simulink model "SunSol_mathBlock"  (R2025b)
settings: Solver=VariableStepAuto  StartTime=0.0  StopTime=10.0  RelTol=1e-3
settings Model: Creator=Abdulwahid  LastModifiedBy=Abdulwahid
settings DataIOCC: SaveOutput=off  SignalLogging=off

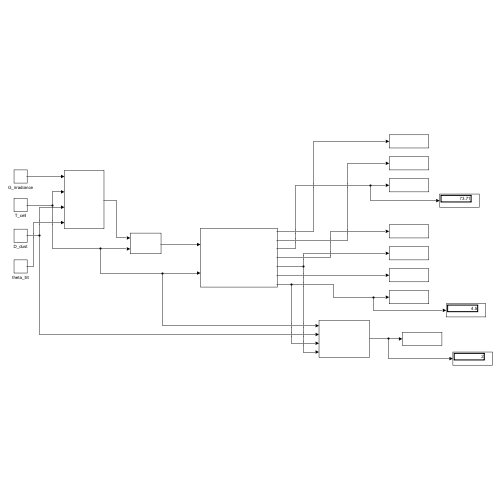
[thumbnail: Simulink's stored preview of the top-level diagram]
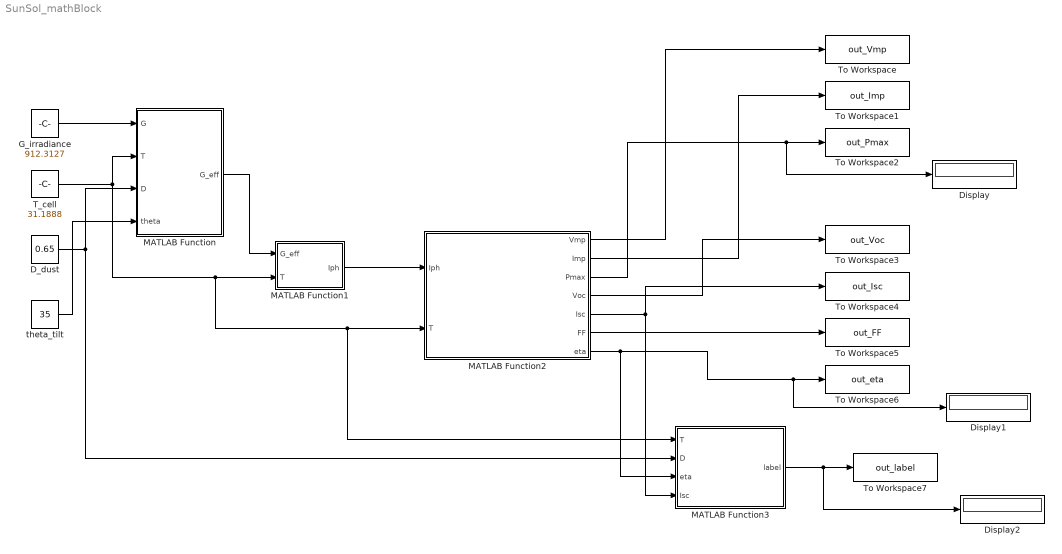
== system SunSol_mathBlock ==
  D_dust : Constant  Value=0.65
  Display : Display
  Display1 : Display
  Display2 : Display
  G_irradiance : Constant  Value=912.3127
  MATLAB Function : MATLAB Function  TreatAsAtomicUnit=on
  MATLAB Function1 : MATLAB Function  TreatAsAtomicUnit=on
  MATLAB Function2 : MATLAB Function  TreatAsAtomicUnit=on
  MATLAB Function3 : MATLAB Function  TreatAsAtomicUnit=on
  T_cell : Constant  Value=31.1888
  To Workspace : ToWorkspace  VariableName=out_Vmp  SampleTime=-1
  To Workspace1 : ToWorkspace  VariableName=out_Imp  SampleTime=-1
  To Workspace2 : ToWorkspace  VariableName=out_Pmax  SampleTime=-1
  To Workspace3 : ToWorkspace  VariableName=out_Voc  SaveFormat=Timeseries  SampleTime=-1
  To Workspace4 : ToWorkspace  VariableName=out_Isc  SampleTime=-1
  To Workspace5 : ToWorkspace  VariableName=out_FF  SampleTime=-1
  To Workspace6 : ToWorkspace  VariableName=out_eta  SampleTime=-1
  To Workspace7 : ToWorkspace  VariableName=out_label  SampleTime=-1
  theta_tilt : Constant  Value=35
  wires:
  G_irradiance/1 -> MATLAB Function/1(G)
  T_cell/1 -> MATLAB Function/2(T), MATLAB Function3/1(T), MATLAB Function2/2(T), MATLAB Function1/2(T)
  MATLAB Function/1(G_eff) -> MATLAB Function1/1(G_eff)
  MATLAB Function1/1(Iph) -> MATLAB Function2/1(Iph)
  MATLAB Function2/1(Vmp) -> To Workspace/1
  MATLAB Function2/2(Imp) -> To Workspace1/1
  MATLAB Function2/3(Pmax) -> Display/1, To Workspace2/1
  MATLAB Function2/4(Voc) -> To Workspace3/1
  MATLAB Function2/5(Isc) -> MATLAB Function3/4(Isc), To Workspace4/1
  MATLAB Function2/6(FF) -> To Workspace5/1
  MATLAB Function2/7(eta) -> MATLAB Function3/3(eta), Display1/1, To Workspace6/1
  MATLAB Function3/1(label) -> Display2/1, To Workspace7/1
  D_dust/1 -> MATLAB Function/3(D), MATLAB Function3/2(D)
  theta_tilt/1 -> MATLAB Function/4(theta)

== matlab function SunSol_mathBlock/MATLAB Function1 ==
  data: G_eff input; Iph output; T input
function Iph = calc_Iph(G_eff, T)
    Isc_ref = 8.91;
    Ki      = 0.0032;
    G_ref   = 1000;
    T_ref   = 25;
    Iph = (Isc_ref + Ki .* (T - T_ref)) .* (G_eff ./ G_ref);
end

== matlab function SunSol_mathBlock/MATLAB Function ==
  data: G input; G_eff output; T input; D input; theta input
function G_eff = calc_Geff(G, T, D, theta)
    G_eff = G .* cosd(theta) .* (1 - D);
end

== matlab function SunSol_mathBlock/MATLAB Function2 ==
  data: Iph input; Vmp output; T input; Imp output; Pmax output; Voc output; Isc output; FF output; eta output
function [Vmp,Imp,Pmax,Voc,Isc,FF,eta] = solve_IV(Iph, T)
    q=1.602e-19; k=1.381e-23; n=1.3;
    A=1.638; Rs=0.221; Rsh=415.405; Ns=60;
    T_ref=25; Kv=-0.0023;
    Tc = T + 273.15;
    Vt = (n*k*Tc*Ns)/q;
    I0_ref = 2.0716e-9;
    I0 = I0_ref*(Tc/(T_ref+273.15))^3 ...
         *exp((q*1.12)/(n*k)*(1/(T_ref+273.15)-1/Tc));
    Voc = Ns*(Vt*log(Iph/I0+1)) + Kv*(T-T_ref);
    Isc = Iph;
    V_arr = linspace(0,Voc,500);
    I_arr = zeros(1,500);
    for i=1:500
        V=V_arr(i); I=Iph;
        for j=1:50
            F  = I-Iph+I0*(exp((V+I*Rs)/Vt)-1)+(V+I*Rs)/Rsh;
            dF = 1+I0*(Rs/Vt)*exp((V+I*Rs)/Vt)+Rs/Rsh;
            I  = I - F/dF;
        end
        I_arr(i)=max(I,0);
    end
    P_arr=V_arr.*I_arr;
    [Pmax,idx]=max(P_arr);
    Vmp=V_arr(idx); Imp=I_arr(idx);
    FF=Pmax/(Voc*Isc);
    eta=(Pmax/(A*1000))*100;
end

== matlab function SunSol_mathBlock/MATLAB Function3 ==
  data: T input; label output; D input; eta input; Isc input
function label = assign_health(T, D, eta, Isc)
    % Use input conditions directly for guaranteed coverage
    % D ranges:     0, 0.129, 0.257, 0.386, 0.514, 0.643, 0.771, 0.9
    % T ranges:     10 to 80
    % Isc proxy for G — low Isc means low G

    Isc_ref = 8.91;
    isHot     = T > 60;
    isDusty   = D > 0.4;
    isShaded  = Isc < 0.4 * Isc_ref;
    isFaulty  = D > 0.7 && Isc < 0.35 * Isc_ref;

    if isFaulty
        label = 5;        % Faulty — extreme dust AND very low light
    elseif isDusty
        label = 2;        % Dusty
    elseif isHot
        label = 3;        % Overheating
    elseif isShaded
        label = 4;        % Shaded
    else
        label = 1;        % Normal
    end
end
